simulink model "ex3_sim1m"  (R2022b)
settings: Solver=ode45  StartTime=0.0  StopTime=2  MaxStep=0.0001  RelTol=1e-3
undefined symbols (not defined in the file): bit, d, denC2, denH, F, mot, numC2, numH, pd, r, rads2rpm, rpm2rads, Ts, umax
settings Model: Creator=loren  LastModifiedBy=loren
settings DataIOCC: ReturnWorkspaceOutputs=off

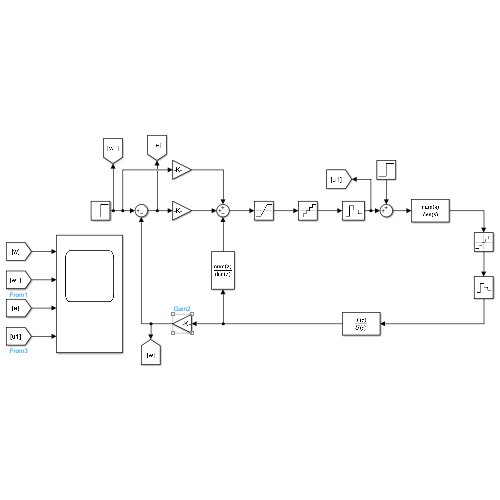
[thumbnail: Simulink's stored preview of the top-level diagram]
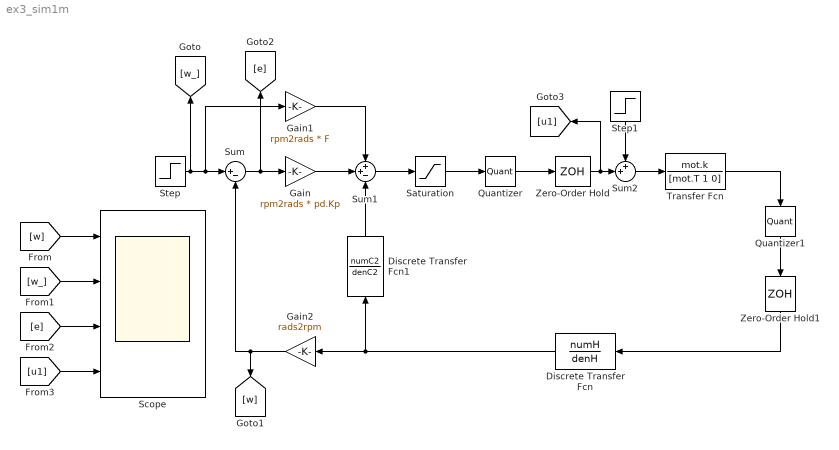
== system ex3_sim1m ==
  Discrete Transfer Fcn : DiscreteTransferFcn  Numerator=numH  Denominator=denH  SampleTime=Ts
  Discrete Transfer Fcn1 : DiscreteTransferFcn  Numerator=numC2  Denominator=denC2  SampleTime=Ts
  Gain : Gain  Gain=rpm2rads * pd.Kp
  Gain1 : Gain  Gain=rpm2rads * F
  Gain2 : Gain  Gain=rads2rpm
  Quantizer : Quantizer  QuantizationInterval=2 * umax / 2^bit
  Quantizer1 : Quantizer  QuantizationInterval=pulse2rad
  Saturation : Saturate  UpperLimit=umax  LowerLimit=-umax
  Scope : Scope  NumInputPorts=4
  Step : Step  Time=r.t  After=r.A  SampleTime=0
  Step1 : Step  Time=d.t  After=d.A  SampleTime=0
  Sum : Sum  Inputs=|+-
  Sum1 : Sum  Inputs=++-
  Sum2 : Sum  Inputs=++|
  Transfer Fcn : TransferFcn  Numerator=mot.k  Denominator=[mot.T 1 0]
  Zero-Order Hold : ZeroOrderHold  SampleTime=Ts
  Zero-Order Hold1 : ZeroOrderHold  SampleTime=Ts
  wires:
  Step/1 -> [w_], Gain1/1, Sum/1
  Sum/1 -> [e], Gain/1
  Gain/1 -> Sum1/2
  Gain1/1 -> Sum1/1
  Sum1/1 -> Saturation/1
  Saturation/1 -> Quantizer/1
  Quantizer/1 -> Zero-Order Hold/1
  Zero-Order Hold/1 -> [u1], Sum2/2
  Sum2/1 -> Transfer Fcn/1
  Step1/1 -> Sum2/1
  Discrete Transfer Fcn1/1 -> Sum1/3
  Discrete Transfer Fcn/1 -> Discrete Transfer Fcn1/1, Gain2/1
  Transfer Fcn/1 -> Quantizer1/1
  Quantizer1/1 -> Zero-Order Hold1/1
  Zero-Order Hold1/1 -> Discrete Transfer Fcn/1
  [u1] -> Scope/4
  [e] -> Scope/3
  [w_] -> Scope/2
  [w] -> Scope/1
  Gain2/1 -> [w], Sum/2
